simulink model "TransferFunction"  (R2020a)
settings: Solver=VariableStepAuto  StartTime=0.0  StopTime=8  RelTol=1e-3
model workspace: external: MATLAB File tfFile.m (data not in the file)
values from neighbouring files (symbols this model uses):
  ETAtot_Kt = 1.8    [tfFile.m]
  Kb = 2    [tfFile.m]
  Kcs = 0.5    [tfFile.m]
  Kf = 0.1    [tfFile.m]
  Kss = 0.0433    [tfFile.m]
  PCwAvor_Itot = 0.6154    [tfFile.m]
  r_Itot = 0.0615    [tfFile.m]
  Ra_inv = 1    [tfFile.m]
libraries: simulink x3
settings Model: OrderedModelArguments=off  Creator=Kimo Store  LastModifiedBy=Kimo Store

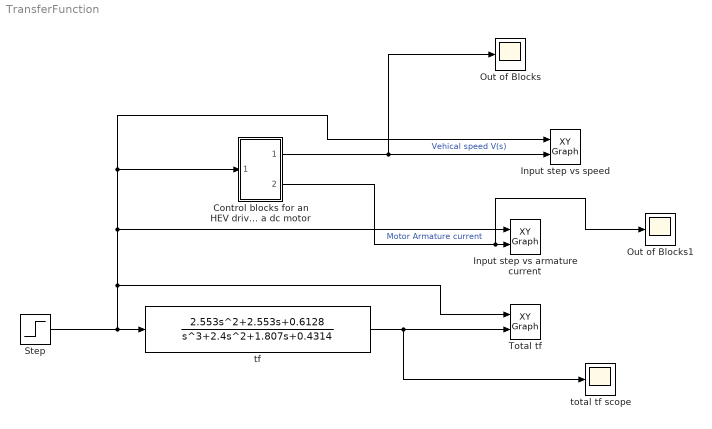
== system TransferFunction ==
  " Control blocks for an HEV driven by a dc motor" : Subsystem
  Input step vs armature current : simulink/Sinks/XY Graph  xmin=-2  xmax=6  ymin=-1  ymax=700  st=-1
  Input step vs speed : simulink/Sinks/XY Graph  xmin=-1  xmax=8  ymin=-8  ymax=8  st=-1
  Out of Blocks : Scope
  Out of Blocks1 : Scope
  Step : Step  After=4  SampleTime=0
  Total tf : simulink/Sinks/XY Graph  xmin=-1  xmax=8  ymin=-8  ymax=8  st=-1
  tf : TransferFcn  Numerator=[2.553 2.553 0.6128]  Denominator=[1 2.4 1.807 0.4314]
      settings: AttributesFormatString=Equivalent transfer function
  total tf scope : Scope
  wires:
  Step/1 -> " Control blocks for an HEV driven by a dc motor"/1(In1), Input step vs speed/1, Input step vs armature current/1, Total tf/1, tf/1
  tf/1 -> total tf scope/1, Total tf/2
  " Control blocks for an HEV driven by a dc motor"/1(Out1) -> Input step vs speed/2, Out of Blocks/1  "Vehical speed V(s)"
  " Control blocks for an HEV driven by a dc motor"/2(Out2) -> Out of Blocks1/1, Input step vs armature current/2  "Motor Armature current"

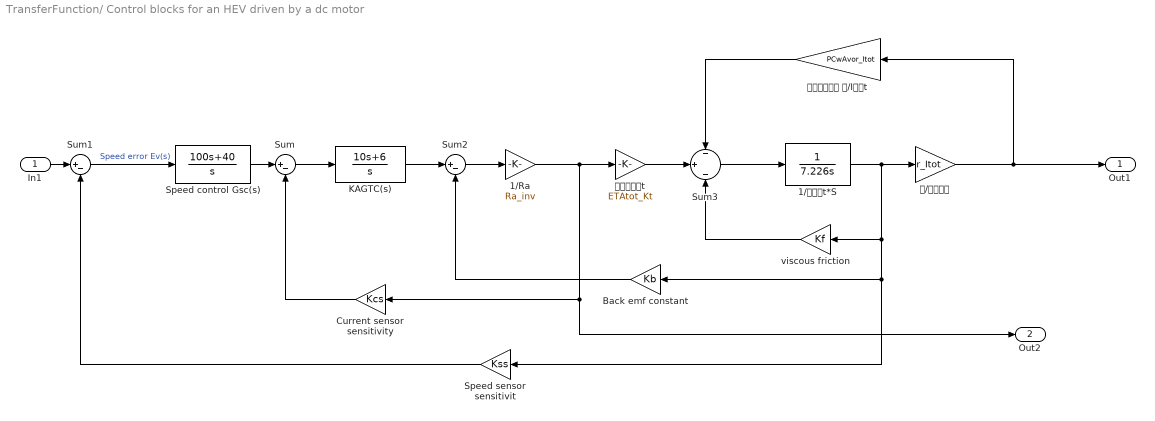
== system TransferFunction/ Control blocks for an HEV driven by a dc motor ==
  In1 : Inport
  1/Ra : Gain  Gain=Ra_inv
      settings: AttributesFormatString=Armature circuit
  1/𝐽𝑡𝑜t*S : TransferFcn  Denominator=[7.226 0]
      settings: AttributesFormatString=Jot is motor inertia
  Back emf constant : Gain  Gain=Kb
  Current sensor sensitivity : Gain  Gain=Kcs
  KAGTC(s) : TransferFcn  Numerator=[10 6]  Denominator=[1 0]
      settings: AttributesFormatString=|
      | Torque controller &
      | power amplifier
  Speed control Gsc(s) : TransferFcn  Numerator=[100 40]  Denominator=[1 0]
  Speed sensor sensitivit : Gain  Gain=Kss
  Sum : Sum  Inputs=|+-
  Sum1 : Sum  Inputs=|+-
  Sum2 : Sum  Inputs=|+-
  Sum3 : Sum  Inputs=-|+|-
  viscous friction : Gain  Gain=Kf
  𝑟/𝑖𝑡𝑜𝑡 : Gain  Gain=r_Itot
      settings: AttributesFormatString=Vehicle dynamics
  𝜂𝑡𝑜𝑡𝐾t : Gain  Gain=ETAtot_Kt
      settings: AttributesFormatString=Motor torque
  𝜌𝑐𝑤𝐴𝑣𝑜 𝑟/I𝑡𝑜t : Gain  Gain=PCwAvor_Itot
      settings: AttributesFormatString=Vehicle dynamics
  Out1 : Outport
  Out2 : Outport  Port=2
  wires:
  1/𝐽𝑡𝑜t*S/1 -> viscous friction/1, Speed sensor sensitivit/1, Back emf constant/1, 𝑟/𝑖𝑡𝑜𝑡/1
  Sum/1 -> KAGTC(s)/1
  Sum3/1 -> 1/𝐽𝑡𝑜t*S/1
  Speed control Gsc(s)/1 -> Sum/1
  In1/1 -> Sum1/1
  1/Ra/1 -> Out2/1, Current sensor sensitivity/1, 𝜂𝑡𝑜𝑡𝐾t/1
  𝜂𝑡𝑜𝑡𝐾t/1 -> Sum3/2
  Sum2/1 -> 1/Ra/1
  𝑟/𝑖𝑡𝑜𝑡/1 -> Out1/1, 𝜌𝑐𝑤𝐴𝑣𝑜 𝑟/I𝑡𝑜t/1
  Current sensor sensitivity/1 -> Sum/2
  KAGTC(s)/1 -> Sum2/1
  𝜌𝑐𝑤𝐴𝑣𝑜 𝑟/I𝑡𝑜t/1 -> Sum3/1
  Speed sensor sensitivit/1 -> Sum1/2
  viscous friction/1 -> Sum3/3
  Back emf constant/1 -> Sum2/2
  Sum1/1 -> Speed control Gsc(s)/1  "Speed error Ev(s)"
